simulink model "TestSoundTone"  (Simulink 6.4)
settings: Solver=FixedStepDiscrete  SolverMode=SingleTasking  StartTime=0  StopTime=inf  FixedStep=0.001  RelTol=1e-3
PreLoadFcn:
  | FrequencyList
values from neighbouring files (symbols this model uses):
  frequency = uint16([33   35   37   39   41   44   46   49   52   55   58   62              65   69   73   78   82   87   92   98  104  110  117  123             131  139  147  156  165  175  185  196  208  220  233  247             262  277  294  311  330  349  370  392  415  440  466  494             523  554  587  622  659  698  740  784  831  880  932  988            1047 1109 1175 1245 1319 1397 1480 1568 ...(+22 chars)    [FrequencyList.m]
libraries: ecrobot_nxt_lib x5
CloseFcn:
  | rtwprivate ssgencode ModelCloseRequest TestBluetooth
settings Model: Creator=tchikama  LastModifiedBy=tchikama  ProdHWDeviceType=ARM7
settings DataIOCC: SaveOutput=off  SignalLogging=off  SaveTime=off
settings OptimizationCC: InlineParams=on  InlineInvariantSignals=on  RollThreshold=2  StateBitsets=on  DataBitsets=on  UseTempVars=on  InitFltsAndDblsToZero=off  NoFixptDivByZeroProtection=on  EfficientFloat2IntCast=on  OptimizeModelRefInitCode=on  LifeSpan=1
settings DebuggingCC: ConsistencyChecking=warning  SignalInfNanChecking=warning  ReadBeforeWriteMsg=DisableAll  WriteAfterWriteMsg=DisableAll  WriteAfterReadMsg=DisableAll  AlgebraicLoopMsg=error  CheckExecutionContextPreStartOutputMsg=on  CheckExecutionContextRuntimeOutputMsg=on  SolverPrmCheckMsg=none  SingleTaskRateTransMsg=warning  TasksWithSamePriorityMsg=none  IntegerOverflowMsg=error  ParameterPrecisionLossMsg=none  UnconnectedInputMsg=error  UnconnectedOutputMsg=error  UnconnectedLineMsg=error  UniqueDataStoreMsg=error  BusObjectLabelMismatch=error  RootOutportRequireBusObject=error  ModelReferenceIOMsg=warning  ModelReferenceVersionMismatchMessage=warning  ModelReferenceIOMismatchMessage=warning
settings HardwareCC: ProdIntDivRoundTo=Zero  ProdEndianess=LittleEndian  ProdHWDeviceType=ARM7  TargetHWDeviceType=32-bit Generic
settings ModelReferenceCC: ModelReferenceNumInstancesAllowed=Single
settings RTWCC: SystemTargetFile=ert.tlc  GenCodeOnly=on  GenerateMakefile=off  TemplateMakefile=ert_default_tmf  Description=Real-Time Workshop Embedded Coder (no auto configuration)  GenerateReport=on  RTWVerbose=off  ProcessScript=ert_make_rtw_hook  IncludeHyperlinkInReport=on  LaunchReport=on
settings CodeAppCC: ForceParamTrailComments=on  IgnoreCustomStorageClasses=off  SFDataObjDesc=on  PrefixModelToSubsysFcnNames=off  CustomSymbolStrGlobalVar=rt$N$M  CustomSymbolStrType=$N$M  CustomSymbolStrFcn=$N$M$F  CustomSymbolStrMacro=$N$M  InsertBlockDesc=on
settings ERTTargetCC: TargetFcnLib=ansi_tfl_tmw.mat  GenFloatMathFcnCalls=GNU  IncludeMdlTerminateFcn=off  SuppressErrorStatus=on  IncludeERTFirstTime=on  SupportAbsoluteTime=off  SupportNonFinite=off  SupportComplex=off  PurelyIntegerCode=on  InlinedParameterPlacement=NonHierarchical  RootIOFormat=Structure reference  ERTCustomFileTemplate=example_file_process.tlc  InitialValueSource=Model

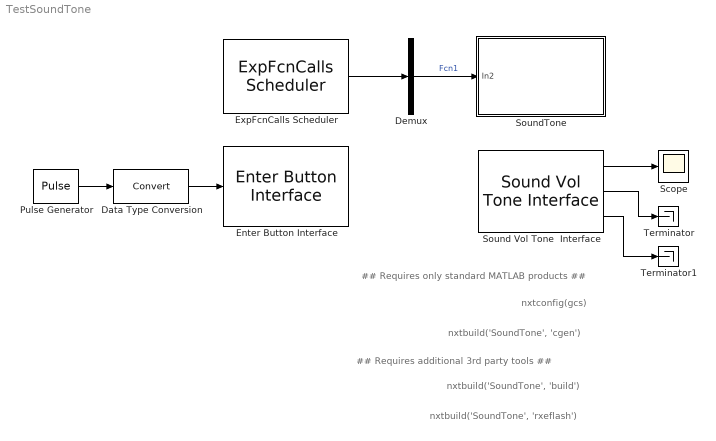
== system TestSoundTone ==
  note: nxtbuild('SoundTone', 'build')
  note: nxtbuild('SoundTone', 'rxeflash')
  note: nxtbuild('SoundTone', 'cgen')
  note: ## Requires only standard MATLAB products ##
  note: ## Requires additional 3rd party tools ##
  note: nxtconfig(gcs)
  Data Type Conversion : DataTypeConversion
  Demux : Demux  Outputs=1
  Enter Button Interface : ecrobot_nxt_lib/Enter Button Interface  SystemSampleTime=-1
  ExpFcnCalls Scheduler : ecrobot_nxt_lib/ExpFcnCalls Scheduler  Priority=1  fcname='Fcn1'  fctrigger=[10]  ts=0.001  platform=OSEK  stacksize=[512]  bd_mode=Slave  bd_addr='00', '16', '53', '04', 'F1', 'B3', '00'
  Pulse Generator : DiscretePulseGenerator  Period=100  PulseWidth=50  SampleTime=0.001
  Scope : Scope
      settings: TimeRange=15  YMin=0  YMax=2500
  Sound Vol Tone  Interface : ecrobot_nxt_lib/Sound Vol Tone  Interface  SystemSampleTime=-1
  SoundTone : Subsystem
  Terminator : Terminator
  Terminator1 : Terminator
  wires:
  ExpFcnCalls Scheduler/1 -> Demux/1
  Pulse Generator/1 -> Data Type Conversion/1
  Demux/1 -> SoundTone/1(In2)  "Fcn1"
  Data Type Conversion/1 -> Enter Button Interface/1
  Sound Vol Tone  Interface/1 -> Scope/1
  Sound Vol Tone  Interface/2 -> Terminator/1
  Sound Vol Tone  Interface/3 -> Terminator1/1

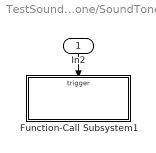
== system TestSoundTone/SoundTone ==
  In2 : Inport  Orientation=down
  Function-Call Subsystem1 : Subsystem  TreatAsAtomicUnit=on
  wires:
  In2/1 -> Function-Call Subsystem1/Trigger

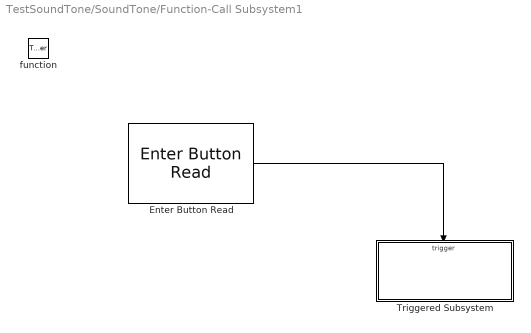
== system TestSoundTone/SoundTone/Function-Call Subsystem1 ==
  function : TriggerPort  TriggerType=function-call
  Enter Button Read : ecrobot_nxt_lib/Enter Button Read  SystemSampleTime=-1
  Triggered Subsystem : Subsystem  TreatAsAtomicUnit=on
  wires:
  Enter Button Read/1 -> Triggered Subsystem/Trigger

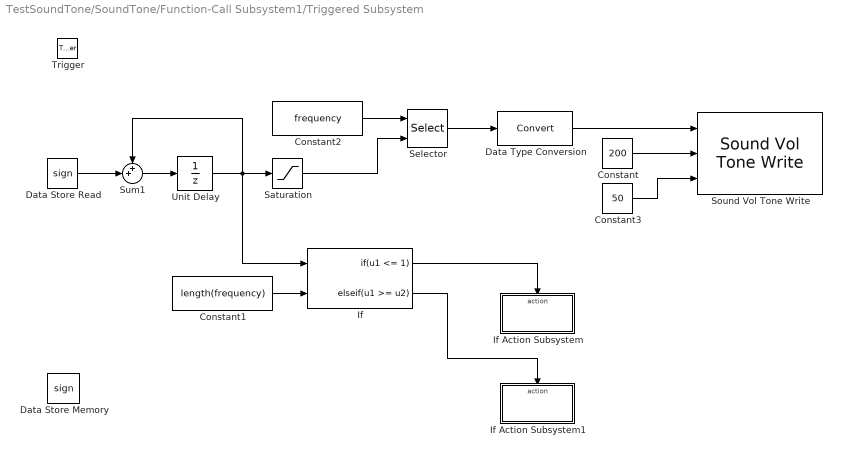
== system TestSoundTone/SoundTone/Function-Call Subsystem1/Triggered Subsystem ==
  Trigger : TriggerPort
  Constant : Constant  Value=200  OutDataType=sfix(16)  ConRadixGroup=Use specified scaling  OutScaling=2^0  SampleTime=inf  FramePeriod=inf
  Constant1 : Constant  Value=length(frequency)  OutDataTypeMode=int32  OutDataType=sfix(16)  ConRadixGroup=Use specified scaling  OutScaling=2^0  SampleTime=inf  FramePeriod=inf
  Constant2 : Constant  Value=frequency  OutDataTypeMode=uint16  OutDataType=sfix(16)  ConRadixGroup=Use specified scaling  OutScaling=2^0  SampleTime=inf  FramePeriod=inf
  Constant3 : Constant  Value=50  OutDataType=sfix(16)  ConRadixGroup=Use specified scaling  OutScaling=2^0  SampleTime=inf  FramePeriod=inf
  Data Store Memory : DataStoreMemory  DataStoreName=sign  ReadBeforeWriteMsg=warning  WriteAfterWriteMsg=warning  WriteAfterReadMsg=warning  InitialValue=1  DataType=int32
  Data Store Read : DataStoreRead  DataStoreName=sign  SampleTime=-1
  Data Type Conversion : DataTypeConversion
  If : If  NumInputs=2  IfExpression=u1 <= 1  ElseIfExpressions=u1 >= u2  ShowElse=off
  If Action Subsystem : Subsystem  TreatAsAtomicUnit=on
  If Action Subsystem1 : Subsystem  TreatAsAtomicUnit=on
  Saturation : Saturate  UpperLimit=length(frequency)  LowerLimit=1
  Selector : Selector  ElementSrc=External  Elements=[1 3]  InputPortWidth=length(frequency)
  Sound Vol Tone Write : ecrobot_nxt_lib/Sound Vol Tone Write
  Sum1 : Sum  Inputs=++|  OutDataTypeMode=int32  InputSameDT=on
  Unit Delay : UnitDelay  X0=1  SampleTime=-1
  wires:
  Unit Delay/1 -> Sum1/1, If/1, Saturation/1
  Constant2/1 -> Selector/1
  Saturation/1 -> Selector/2
  Selector/1 -> Data Type Conversion/1
  Sum1/1 -> Unit Delay/1
  Data Store Read/1 -> Sum1/2
  Constant1/1 -> If/2
  If/1 -> If Action Subsystem/Action
  If/2 -> If Action Subsystem1/Action
  Data Type Conversion/1 -> Sound Vol Tone Write/1
  Constant/1 -> Sound Vol Tone Write/2
  Constant3/1 -> Sound Vol Tone Write/3

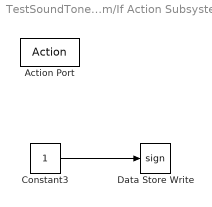
== system TestSoundTone/SoundTone/Function-Call Subsystem1/Triggered Subsystem/If Action Subsystem ==
  Action Port : ActionPort  ActionType=then
  Constant3 : Constant  Value=1  OutDataTypeMode=int32  OutDataType=sfix(16)  ConRadixGroup=Use specified scaling  OutScaling=2^0  SampleTime=inf  FramePeriod=inf
  Data Store Write : DataStoreWrite  DataStoreName=sign  SampleTime=-1
  wires:
  Constant3/1 -> Data Store Write/1

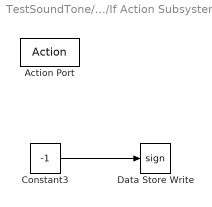
== system TestSoundTone/SoundTone/Function-Call Subsystem1/Triggered Subsystem/If Action Subsystem1 ==
  Action Port : ActionPort  ActionType=elseif
  Constant3 : Constant  Value=-1  OutDataTypeMode=int32  OutDataType=sfix(16)  ConRadixGroup=Use specified scaling  OutScaling=2^0  SampleTime=inf  FramePeriod=inf
  Data Store Write : DataStoreWrite  DataStoreName=sign  SampleTime=-1
  wires:
  Constant3/1 -> Data Store Write/1
